simulink model "SIM_VELOCIDAD"  (R2021a)
settings: Solver=ode3  StartTime=0.0  StopTime=Velocidad(end,1)-Velocidad(1,1)  FixedStep=tr  MaxStep=tc  RelTol=1e-6  AbsTol=1e-9
InitFcn:
  | % Periodo de muestreo control
  | ts=20e-3;
  | % Periodo de muestreo registro
  | tr=5e-3;
  | % Constante de tiempo de filtrado
  | Tf_vel=200e-3; % Velocidad
values from neighbouring files (symbols this model uses):
  K = mu*Kp    [ControlP.m]    (also in ControlPID_RF.m)
  Km = 0.077871    [ControlP.m]    (also in ControlPID_RF.m)
  N = (1/(mu*f))-1    [ControlP.m]    (also in ControlPID_RF.m)
  Td = ((1/mu)-f)*D    [ControlP.m]    (also in ControlPID_RF.m)
  Ti = mu*I    [ControlP.m]    (also in ControlPID_RF.m)
  Tm = 0.067567    [ControlP.m]    (also in ControlPID_RF.m)
undefined symbols (not defined in the file or in its folder): DiscIntNeverNeededParam
libraries: simulink x3
settings Model: ExtModeTrigMode=oneshot  ExtModeArmWhenConnect=off  Creator=zamora  LastModifiedBy=ferna
settings SolverCC: AutoScaleAbsTol=off  AlgebraicLoopSolver=TrustRegion
settings DataIOCC: SaveFormat=Array  SignalLoggingSaveFormat=ModelDataLogs  SaveOutput=off  SaveTime=off  ReturnWorkspaceOutputs=off  StateSaveName=x  TimeSaveName=t  OutputSaveName=y
settings OptimizationCC: BlockReduction=off  BooleanDataType=off  DefaultParameterBehavior=Inlined  BufferReuse=off  ExpressionDepthLimit=2147483647  LifeSpan=inf
settings DebuggingCC: SaveWithParameterizedLinksMsg=none  UnderspecifiedInitializationDetection=Classic  MergeDetectMultiDrivingBlocksExec=none  SignalResolutionControl=TryResolveAllWithWarning  MultiTaskDSMMsg=warning  MultiTaskCondExecSysMsg=none  ParameterPrecisionLossMsg=none  FcnCallInpInsideContextMsg=warning  StateNameClashWarn=warning  InitInArrayFormatMsg=none  SFUnexpectedBacktrackingDiag=warning  SFNoUnconditionalDefaultTransitionDiag=warning  SFExecutionAtInitializationDiag=none  SFMachineParentedDataDiag=warning  ArithmeticOperatorsInVariantConditions=warning
settings HardwareCC: ProdBitPerPointer=32  ProdBitPerSizeT=32  ProdBitPerPtrDiffT=32  ProdLargestAtomicFloat=None  ProdIntDivRoundTo=Undefined  ProdEndianess=Unspecified  ProdWordSize=32  ProdHWDeviceType=32-bit Generic  TargetBitPerPointer=64  TargetBitPerSizeT=64  TargetBitPerPtrDiffT=64  TargetLongLongMode=on  TargetIntDivRoundTo=Zero  TargetEndianess=LittleEndian  TargetWordSize=64  TargetHWDeviceType=MATLAB Host  ProdEqTarget=off
settings ModelReferenceCC: PropagateSignalLabelsOutOfModel=off
settings SFSimCC: SimUseLocalCustomCode=off  CustomCodeUndefinedFunction=UseInterfaceOnly
settings RTWCC: TemplateMakefile=grt_unix.tmf  RTWUseLocalCustomCode=off
settings CodeAppCC: StateflowObjectComments=on
settings GRTTargetCC: TargetLangStandard=C89/C90 (ANSI)  CombineOutputUpdateFcns=off  GRTInterface=on
settings ConfigComp: CovMetricSettings=dw  CovSaveCumulativeToWorkspaceVar=on  CovSaveSingleToWorkspaceVar=on  CovExternalEMLEnable=off  CovSFcnEnable=off

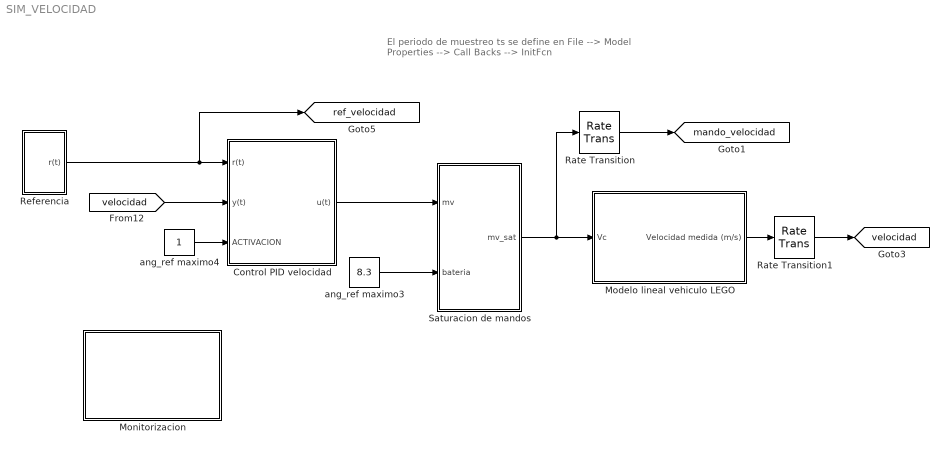
== system SIM_VELOCIDAD ==
  note: El periodo de muestreo ts se define en
      | File --> Model Properties --> Call Backs --> InitFcn
  Control PID velocidad : Subsystem  mask{K=K, Ti=Ti, Td=Td, N=N, b=1, ts=ts}
      mask init:
      | %%%%%%%%%%%%%%%%%%%%%%%%%%%%%%%%%%%%%%%%%%%%%%
      | %  DISCRETIZACION DE LA ACCION DIFERENCIAL
      | %%%%%%%%%%%%%%%%%%%%%%%%%%%%%%%%%%%%%%%%%%%%%%
      | z=tf('z',ts);
      | sa=2*(1-z^-1)/ts/(1+z^-1); % Derivada en retraso
      | AD=Td*sa/(1+Td/N*sa);
  Modelo lineal vehiculo LEGO : Subsystem  mask{Km_v=Km, Tm_v=Tm, Tr=0.571063329995719}
      mask prompts: Km_v "Ganancia velocidad"; Tm_v "Constante de tiempo velocidad"; Tr "Par resistente equivalente (V)"
  Monitorizacion : Subsystem
  Rate Transition : RateTransition  OutPortSampleTime=tr
  Rate Transition1 : RateTransition  OutPortSampleTime=tr
  Referencia : Subsystem
  Saturacion de mandos : Subsystem
  ang_ref maximo3 : Constant  Value=8.3  OutDataTypeStr=double  SampleTime=ts
  ang_ref maximo4 : Constant  OutDataTypeStr=single  SampleTime=ts
  tag scope: mando_velocidad=global, ref_velocidad=global, velocidad=global
  wires:
  Modelo lineal vehiculo LEGO/1(Velocidad medida (m/s)) -> Rate Transition1/1
  Saturacion de mandos/1(mv_sat) -> Modelo lineal vehiculo LEGO/1(Vc), Rate Transition/1
  [velocidad] -> Control PID velocidad/2(y(t))
  Referencia/1(r(t)) -> Control PID velocidad/1(r(t)), [ref_velocidad]
  ang_ref maximo3/1 -> Saturacion de mandos/2(bateria)
  Control PID velocidad/1(u(t)) -> Saturacion de mandos/1(mv)
  ang_ref maximo4/1 -> Control PID velocidad/3(ACTIVACION)
  Rate Transition/1 -> [mando_velocidad]
  Rate Transition1/1 -> [velocidad]

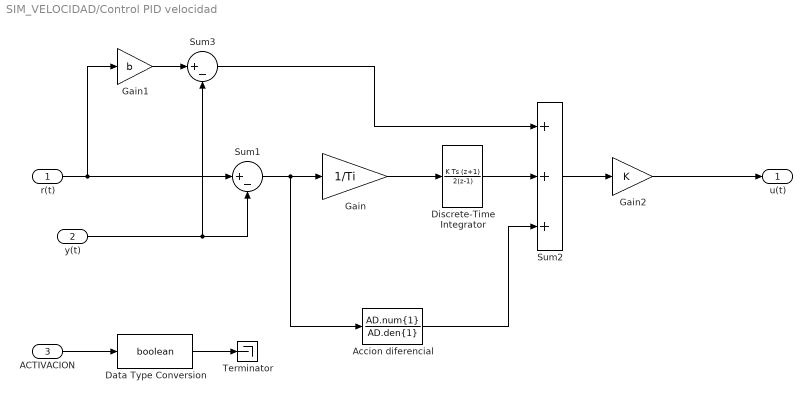
== system SIM_VELOCIDAD/Control PID velocidad ==
  r(t) : Inport  SampleTime=ts
  y(t) : Inport  Port=2  SampleTime=ts
  ACTIVACION : Inport  Port=3  SampleTime=ts
  Accion diferencial : DiscreteTransferFcn  Numerator=AD.num{1}  Denominator=AD.den{1}  SampleTime=ts
  Data Type Conversion : DataTypeConversion  OutDataTypeStr=boolean
  Discrete-Time Integrator : DiscreteIntegrator  IntegratorMethod=Integration: Trapezoidal  SampleTime=ts  ICPrevOutput=DiscIntNeverNeededParam  ICPrevScaledInput=DiscIntNeverNeededParam
  Gain : Gain  Gain=1/Ti
  Gain1 : Gain  Gain=b
  Gain2 : Gain  Gain=K  SampleTime=ts
  Sum1 : Sum  Inputs=|+-
  Sum2 : Sum  Inputs=+++
  Sum3 : Sum  Inputs=|+-
  Terminator : Terminator
  u(t) : Outport  VectorParamsAs1DForOutWhenUnconnected=off
  wires:
  Gain2/1 -> u(t)/1
  ACTIVACION/1 -> Data Type Conversion/1
  y(t)/1 -> Sum3/2, Sum1/2
  r(t)/1 -> Sum1/1, Gain1/1
  Sum1/1 -> Accion diferencial/1, Gain/1
  Sum2/1 -> Gain2/1
  Discrete-Time Integrator/1 -> Sum2/2
  Gain/1 -> Discrete-Time Integrator/1
  Sum3/1 -> Sum2/1
  Gain1/1 -> Sum3/1
  Accion diferencial/1 -> Sum2/3
  Data Type Conversion/1 -> Terminator/1

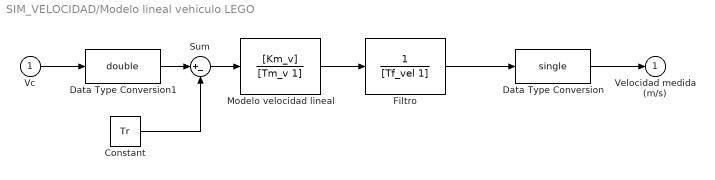
== system SIM_VELOCIDAD/Modelo lineal vehiculo LEGO ==
  Vc : Inport
  Constant : Constant  Value=Tr  SampleTime=0
  Data Type Conversion : DataTypeConversion  OutDataTypeStr=single
  Data Type Conversion1 : DataTypeConversion  OutDataTypeStr=double
  Filtro : TransferFcn  Numerator=1  Denominator=[Tf_vel 1]
  Modelo velocidad lineal : TransferFcn  Numerator=[Km_v]  Denominator=[Tm_v 1]
  Sum : Sum  Inputs=|+-
  Velocidad medida (m/s) : Outport  OutDataTypeStr=single  InitialOutput=0  VectorParamsAs1DForOutWhenUnconnected=off
  wires:
  Modelo velocidad lineal/1 -> Filtro/1
  Filtro/1 -> Data Type Conversion/1
  Vc/1 -> Data Type Conversion1/1
  Data Type Conversion/1 -> Velocidad medida (m/s)/1
  Data Type Conversion1/1 -> Sum/1
  Sum/1 -> Modelo velocidad lineal/1
  Constant/1 -> Sum/2

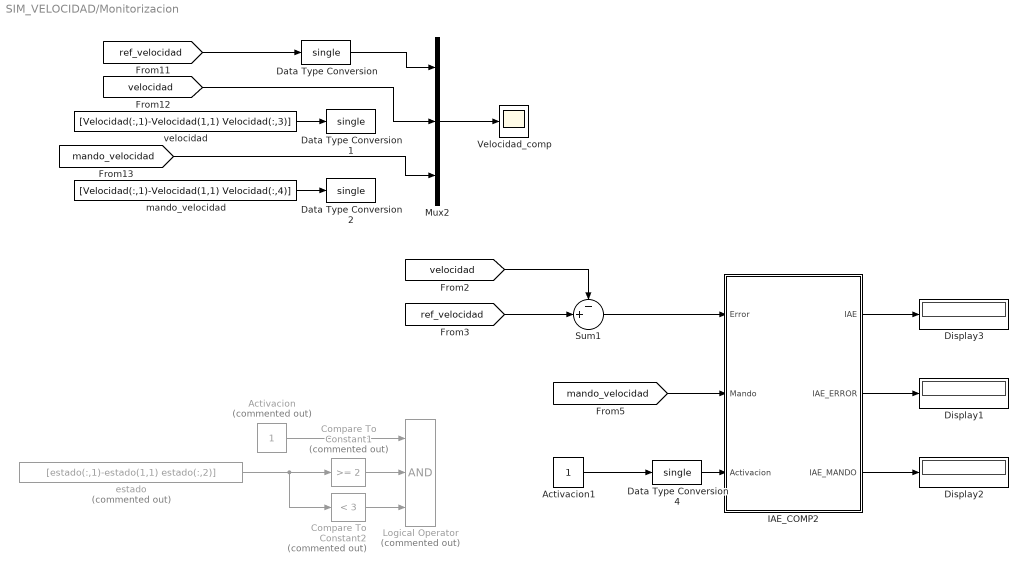
== system SIM_VELOCIDAD/Monitorizacion ==
  Activacion : Constant  Commented=on  SampleTime=tr
  Activacion1 : Constant  SampleTime=tr
  Compare To Constant1 : simulink/Logic and Bit Operations/Compare To Constant  Commented=on  relop=>=  const=2  OutDataTypeStr=uint8
  Compare To Constant2 : simulink/Logic and Bit Operations/Compare To Constant  Commented=on  relop=<  const=3  OutDataTypeStr=uint8
  Data Type Conversion{,1..2,4} (4 alike) : DataTypeConversion  OutDataTypeStr=single
  Display1 : Display
      settings: Decimation=50
  Display2 : Display
      settings: Decimation=50
  Display3 : Display
      settings: Decimation=50
  IAE_COMP2 : Subsystem
      mask init:
      | SCALE = 300000;
      | FACTOR_MANDO = 2.5e-3;
  Logical Operator : Logic  Commented=on  Inputs=3  AllPortsSameDT=off  OutDataTypeStr=boolean
  Mux2 : Mux  Inputs=3
  Sum1 : Sum  Inputs=-+|  SampleTime=tr
  Velocidad_comp : Scope
  estado : FromWorkspace  Commented=on  VariableName=[estado(:,1)-estado(1,1) estado(:,2)]  SampleTime=tr
  "mando_velocidad " : FromWorkspace  VariableName=[Velocidad(:,1)-Velocidad(1,1) Velocidad(:,4)]  SampleTime=tr
  velocidad : FromWorkspace  VariableName=[Velocidad(:,1)-Velocidad(1,1) Velocidad(:,3)]  SampleTime=tr
  wires:
  [ref_velocidad] -> Data Type Conversion/1
  Mux2/1 -> Velocidad_comp/1
  [velocidad] -> Mux2/2
  velocidad/1 -> Data Type Conversion1/1
  "mando_velocidad "/1 -> Data Type Conversion2/1
  Data Type Conversion/1 -> Mux2/1
  Data Type Conversion4/1 -> IAE_COMP2/3(Activacion)
  Sum1/1 -> IAE_COMP2/1(Error)
  [ref_velocidad] -> Sum1/2
  [velocidad] -> Sum1/1
  [mando_velocidad] -> IAE_COMP2/2(Mando)
  IAE_COMP2/1(IAE) -> Display3/1
  IAE_COMP2/2(IAE_ERROR) -> Display1/1
  IAE_COMP2/3(IAE_MANDO) -> Display2/1
  Compare To Constant1/1 -> Logical Operator/2
  Compare To Constant2/1 -> Logical Operator/3
  estado/1 -> Compare To Constant2/1, Compare To Constant1/1
  Activacion/1 -> Logical Operator/1
  Activacion1/1 -> Data Type Conversion4/1
  [mando_velocidad] -> Mux2/3

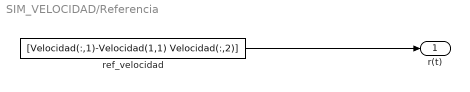
== system SIM_VELOCIDAD/Referencia ==
  ref_velocidad : FromWorkspace  VariableName=[Velocidad(:,1)-Velocidad(1,1) Velocidad(:,2)]  SampleTime=tr
  r(t) : Outport  VectorParamsAs1DForOutWhenUnconnected=off
  wires:
  ref_velocidad/1 -> r(t)/1

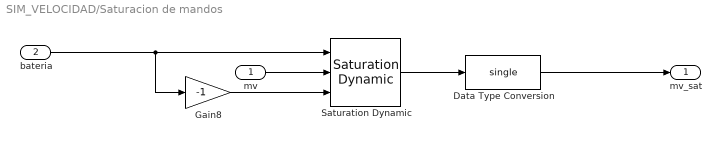
== system SIM_VELOCIDAD/Saturacion de mandos ==
  mv : Inport
  bateria : Inport  Port=2  SampleTime=ts
  Data Type Conversion : DataTypeConversion  OutDataTypeStr=single
  Gain8 : Gain  Gain=-1
  Saturation Dynamic : simulink/Discontinuities/Saturation Dynamic  OutMin=[]  OutMax=[]  OutDataTypeStr=Inherit: Same as second input  OutDataType=fixdt(1, 16)  OutScaling=2^-10  DoSatur=off
  mv_sat : Outport  VectorParamsAs1DForOutWhenUnconnected=off
  wires:
  Gain8/1 -> Saturation Dynamic/3
  bateria/1 -> Gain8/1, Saturation Dynamic/1
  mv/1 -> Saturation Dynamic/2
  Saturation Dynamic/1 -> Data Type Conversion/1
  Data Type Conversion/1 -> mv_sat/1

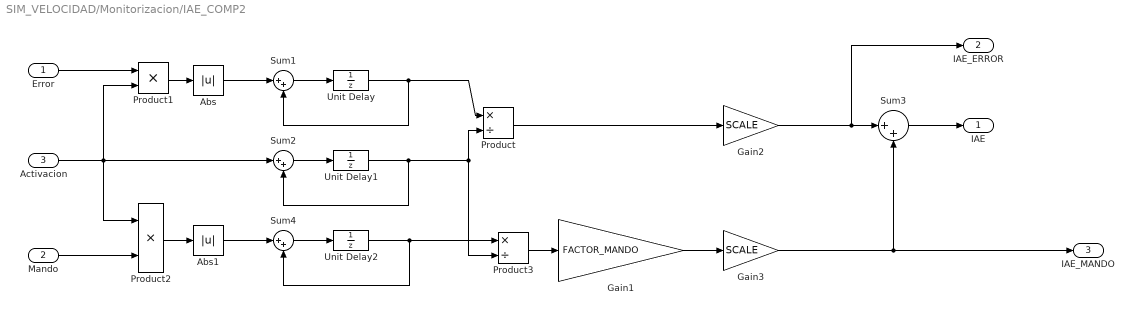
== system SIM_VELOCIDAD/Monitorizacion/IAE_COMP2 ==
  Error : Inport
  Mando : Inport  Port=2
  Activacion : Inport  Port=3
  Abs : Abs
  Abs1 : Abs
  Gain1 : Gain  Gain=FACTOR_MANDO
  Gain2 : Gain  Gain=SCALE
  Gain3 : Gain  Gain=SCALE
  Product : Product  Inputs=*/  RndMeth=Zero
  Product1 : Product  RndMeth=Zero
  Product2 : Product  RndMeth=Zero
  Product3 : Product  Inputs=*/  RndMeth=Zero
  Sum1 : Sum  Inputs=|++
  Sum2 : Sum  Inputs=|++
  Sum3 : Sum  Inputs=|++  SampleTime=tr
  Sum4 : Sum  Inputs=|++
  Unit Delay : UnitDelay  SampleTime=-1  HasFrameUpgradeWarning=on
  Unit Delay1 : UnitDelay  InitialCondition=1  SampleTime=-1  HasFrameUpgradeWarning=on
  Unit Delay2 : UnitDelay  SampleTime=-1  HasFrameUpgradeWarning=on
  IAE : Outport  VectorParamsAs1DForOutWhenUnconnected=off
  IAE_ERROR : Outport  Port=2  VectorParamsAs1DForOutWhenUnconnected=off
  IAE_MANDO : Outport  Port=3  VectorParamsAs1DForOutWhenUnconnected=off
  wires:
  Product3/1 -> Gain1/1
  Abs1/1 -> Sum4/1
  Sum4/1 -> Unit Delay2/1
  Unit Delay2/1 -> Sum4/2, Product3/1
  Mando/1 -> Product2/2
  Product2/1 -> Abs1/1
  Gain3/1 -> IAE_MANDO/1, Sum3/2
  Gain2/1 -> Sum3/1, IAE_ERROR/1
  Gain1/1 -> Gain3/1
  Product/1 -> Gain2/1
  Sum3/1 -> IAE/1
  Abs/1 -> Sum1/1
  Sum1/1 -> Unit Delay/1
  Unit Delay/1 -> Sum1/2, Product/1
  Sum2/1 -> Unit Delay1/1
  Unit Delay1/1 -> Sum2/2, Product/2, Product3/2
  Activacion/1 -> Sum2/1, Product1/2, Product2/1
  Product1/1 -> Abs/1
  Error/1 -> Product1/1
